simulink model "PubIfDecisionLSM_MDL"  (R2020b)
settings: configuration reference "DspaceConfig" (kept outside this file)
PostLoadFcn:
  | if any(exist('dsrtsu_mdlpostloadfcn', 'file') ~= 0), dsrtsu_mdlpostloadfcn('Execute', bdroot); end
InitFcn:
  | , if any(exist('rtifpga_mdlclblib', 'file') ~= 0), rtifpga_mdlclblib('Init', bdroot); end,
  | , if any(exist('dsmpb_private', 'file') ~= 0), dsmpb_private('dsmpb_mdlclblib', 'Init', bdroot); end,
values from neighbouring files (symbols this model uses):
  P_LSM_ALC_Enable = 0.0    [LSM_Parameter.sldd]
  P_LSM_AwayEdge_offset = 0.1    [LSM_Parameter.sldd]
  P_LSM_CentValidErr = 1.0    [LSM_Parameter.sldd]
  P_LSM_DOP_C0_EN_Limit = 0.8    [LSM_Parameter.sldd]
  P_LSM_DOP_C0_out_Limit = 2.0    [LSM_Parameter.sldd]
  P_LSM_DOP_C1_EN_Limit : value not decoded    [LSM_Parameter.sldd]
  P_LSM_DOP_C1_out_Limit : value not decoded    [LSM_Parameter.sldd]
  P_LSM_DOP_C1AndC2_Lim_X : value not decoded    [LSM_Parameter.sldd]
  P_LSM_DOP_C2_EN_Limit : value not decoded    [LSM_Parameter.sldd]
  P_LSM_DOP_C2_out_Limit : value not decoded    [LSM_Parameter.sldd]
  P_LSM_DOP_In_Pre2Dop_Dis = 1.0    [LSM_Parameter.sldd]
  P_LSM_DOP_Out_Pre2Dop_Dis = 2.0    [LSM_Parameter.sldd]
  P_LSM_DOP_PreDis_X : value not decoded    [LSM_Parameter.sldd]
  P_LSM_DOP_PreDis_Y : value not decoded    [LSM_Parameter.sldd]
  P_LSM_DOPEnableSW = 1.0    [LSM_Parameter.sldd]
  P_LSM_DOPValid_CheckTime = 0.06    [LSM_Parameter.sldd]
  P_LSM_DoubleLine_Curr2Cent_Dislimit = 0.5    [LSM_Parameter.sldd]
  P_LSM_DoubleLine_Dop2Cent_Dislimit = 0.5    [LSM_Parameter.sldd]
  P_LSM_DoubleLine_DOPOut_C1 : value not decoded    [LSM_Parameter.sldd]
  P_LSM_DoubleLine_Pre2Cent_Dislimit = 1.0    [LSM_Parameter.sldd]
  P_LSM_Error_Limit = 0.5    [LSM_Parameter.sldd]
  P_LSM_IFV2CenterAxis = 0.0    [LSM_Parameter.sldd]
  P_LSM_IFV2RearAxis = 0.0    [LSM_Parameter.sldd]
  P_LSM_Line2Edge_limit = 0.5    [LSM_Parameter.sldd]
  P_LSM_Line_Error = 0.1    [LSM_Parameter.sldd]
  P_LSM_LineSTD_Limit = 0.15    [LSM_Parameter.sldd]
  P_LSM_NOH_Switch = 0.0    [LSM_Parameter.sldd]
  P_LSM_OTL_C0_Factor = 1.0    [LSM_Parameter.sldd]
  P_LSM_OTL_C1_Factor = 0.5    [LSM_Parameter.sldd]
  P_LSM_OTL_C2_Factor = 0.5    [LSM_Parameter.sldd]
  P_LSM_Pre2OnlyLineDis = 5.0    [LSM_Parameter.sldd]
  P_LSM_Pre_t = 0.0    [LSM_Parameter.sldd]
  P_LSM_SingleLine_Cent2Edge_Dislimit = 100.0    [LSM_Parameter.sldd]
  P_LSM_SingleLine_Curr2Cent_Dislimit = 0.2    [LSM_Parameter.sldd]
  P_LSM_SingleLine_Dop2Cent_Dislimit = 0.2    [LSM_Parameter.sldd]
  P_LSM_SingleLine_DOPOut_C1 : value not decoded    [LSM_Parameter.sldd]
  P_LSM_SingleLine_Pre2Cent_Dislimit = 0.5    [LSM_Parameter.sldd]
  P_LSM_TJALimitSpd = 60.0    [LSM_Parameter.sldd]
undefined symbols (not defined in the file or in its folder): P_lCS_IFV2CenterAxis, P_LCS_IFV2RearAxis, P_LSM_EntryEdge_offset, P_LSM_EntryLnChngEnSwitch, P_LSM_EntryVanishDis, P_LSM_LinetLostTime, P_LSM_LineWijCal_C12, P_LSM_LineWijCal_C13, P_LSM_MapValid_ErrorSwitch, P_LSM_PosLineLcFac, P_LSM_SpdLim_Stub_Spd, P_LSM_SpdLim_StubLength, P_LSM_SpdTurnAlarm
libraries: simulink x324, TrueDurationTime x11
(part 14 of 25)

== system PubIfDecisionLSM_MDL/Subsystem1/TargetLineCalc_20ms/TargetLineCalc/Subsystem3/Subsystem2/Subsystem10 ==
  u : Inport
  MATLAB Function14 : MATLAB Function  TreatAsAtomicUnit=on
  Unit Delay : UnitDelay  SampleTime=-1  HasFrameUpgradeWarning=on
  y : Outport
  wires:
  MATLAB Function14/2(i) -> Unit Delay/1
  u/1 -> MATLAB Function14/1(u)
  Unit Delay/1 -> MATLAB Function14/2(i_k)
  MATLAB Function14/1(y) -> y/1

== system PubIfDecisionLSM_MDL/Subsystem1/TargetLineCalc_20ms/TargetLineCalc/Subsystem3/Subsystem2/Subsystem11 ==
  u : Inport
  MATLAB Function14 : MATLAB Function  TreatAsAtomicUnit=on
  Unit Delay : UnitDelay  SampleTime=-1  HasFrameUpgradeWarning=on
  y : Outport
  wires:
  MATLAB Function14/1(y) -> y/1
  Unit Delay/1 -> MATLAB Function14/2(i_k)
  u/1 -> MATLAB Function14/1(u)
  MATLAB Function14/2(i) -> Unit Delay/1

== system PubIfDecisionLSM_MDL/Subsystem1/TargetLineCalc_20ms/TargetLineCalc/Subsystem3/Subsystem2/Subsystem12 ==
  u : Inport
  MATLAB Function14 : MATLAB Function  TreatAsAtomicUnit=on
  Unit Delay : UnitDelay  SampleTime=-1  HasFrameUpgradeWarning=on
  y : Outport
  wires:
  MATLAB Function14/2(i) -> Unit Delay/1
  u/1 -> MATLAB Function14/1(u)
  Unit Delay/1 -> MATLAB Function14/2(i_k)
  MATLAB Function14/1(y) -> y/1

== system PubIfDecisionLSM_MDL/Subsystem1/TargetLineCalc_20ms/TargetLineCalc/Subsystem3/Subsystem2/Subsystem13 ==
  u : Inport
  MATLAB Function14 : MATLAB Function  TreatAsAtomicUnit=on
  Unit Delay : UnitDelay  SampleTime=-1  HasFrameUpgradeWarning=on
  y : Outport
  wires:
  MATLAB Function14/2(i) -> Unit Delay/1
  u/1 -> MATLAB Function14/1(u)
  Unit Delay/1 -> MATLAB Function14/2(i_k)
  MATLAB Function14/1(y) -> y/1

== system PubIfDecisionLSM_MDL/Subsystem1/TargetLineCalc_20ms/TargetLineCalc/Subsystem3/Subsystem2/Subsystem14 ==
  u : Inport
  MATLAB Function14 : MATLAB Function  TreatAsAtomicUnit=on
  Unit Delay : UnitDelay  SampleTime=-1  HasFrameUpgradeWarning=on
  y : Outport
  wires:
  MATLAB Function14/1(y) -> y/1
  Unit Delay/1 -> MATLAB Function14/2(i_k)
  u/1 -> MATLAB Function14/1(u)
  MATLAB Function14/2(i) -> Unit Delay/1

== system PubIfDecisionLSM_MDL/Subsystem1/TargetLineCalc_20ms/TargetLineCalc/Subsystem3/Subsystem2/Subsystem15 ==
  u : Inport
  MATLAB Function14 : MATLAB Function  TreatAsAtomicUnit=on
  Unit Delay : UnitDelay  SampleTime=-1  HasFrameUpgradeWarning=on
  y : Outport
  wires:
  MATLAB Function14/1(y) -> y/1
  Unit Delay/1 -> MATLAB Function14/2(i_k)
  u/1 -> MATLAB Function14/1(u)
  MATLAB Function14/2(i) -> Unit Delay/1

== system PubIfDecisionLSM_MDL/Subsystem1/TargetLineCalc_20ms/TargetLineCalc/Subsystem3/Subsystem2/Subsystem16 ==
  u : Inport
  MATLAB Function14 : MATLAB Function  TreatAsAtomicUnit=on
  Unit Delay : UnitDelay  SampleTime=-1  HasFrameUpgradeWarning=on
  y : Outport
  wires:
  MATLAB Function14/2(i) -> Unit Delay/1
  u/1 -> MATLAB Function14/1(u)
  Unit Delay/1 -> MATLAB Function14/2(i_k)
  MATLAB Function14/1(y) -> y/1

== system PubIfDecisionLSM_MDL/Subsystem1/TargetLineCalc_20ms/TargetLineCalc/Subsystem3/Subsystem2/Subsystem2 ==
  u : Inport
  MATLAB Function14 : MATLAB Function  TreatAsAtomicUnit=on
  Unit Delay : UnitDelay  SampleTime=-1  HasFrameUpgradeWarning=on
  y : Outport
  wires:
  MATLAB Function14/1(y) -> y/1
  Unit Delay/1 -> MATLAB Function14/2(i_k)
  u/1 -> MATLAB Function14/1(u)
  MATLAB Function14/2(i) -> Unit Delay/1

== system PubIfDecisionLSM_MDL/Subsystem1/TargetLineCalc_20ms/TargetLineCalc/Subsystem3/Subsystem2/Subsystem3 ==
  u : Inport
  MATLAB Function14 : MATLAB Function  TreatAsAtomicUnit=on
  Unit Delay : UnitDelay  SampleTime=-1  HasFrameUpgradeWarning=on
  y : Outport
  wires:
  MATLAB Function14/2(i) -> Unit Delay/1
  u/1 -> MATLAB Function14/1(u)
  Unit Delay/1 -> MATLAB Function14/2(i_k)
  MATLAB Function14/1(y) -> y/1

== system PubIfDecisionLSM_MDL/Subsystem1/TargetLineCalc_20ms/TargetLineCalc/Subsystem3/Subsystem2/Subsystem4 ==
  u : Inport
  MATLAB Function14 : MATLAB Function  TreatAsAtomicUnit=on
  Unit Delay : UnitDelay  SampleTime=-1  HasFrameUpgradeWarning=on
  y : Outport
  wires:
  MATLAB Function14/1(y) -> y/1
  Unit Delay/1 -> MATLAB Function14/2(i_k)
  u/1 -> MATLAB Function14/1(u)
  MATLAB Function14/2(i) -> Unit Delay/1

== system PubIfDecisionLSM_MDL/Subsystem1/TargetLineCalc_20ms/TargetLineCalc/Subsystem3/Subsystem2/Subsystem5 ==
  u : Inport
  MATLAB Function14 : MATLAB Function  TreatAsAtomicUnit=on
  Unit Delay : UnitDelay  SampleTime=-1  HasFrameUpgradeWarning=on
  y : Outport
  wires:
  MATLAB Function14/1(y) -> y/1
  Unit Delay/1 -> MATLAB Function14/2(i_k)
  u/1 -> MATLAB Function14/1(u)
  MATLAB Function14/2(i) -> Unit Delay/1

== system PubIfDecisionLSM_MDL/Subsystem1/TargetLineCalc_20ms/TargetLineCalc/Subsystem3/Subsystem2/Subsystem6 ==
  u : Inport
  MATLAB Function14 : MATLAB Function  TreatAsAtomicUnit=on
  Unit Delay : UnitDelay  SampleTime=-1  HasFrameUpgradeWarning=on
  y : Outport
  wires:
  MATLAB Function14/2(i) -> Unit Delay/1
  u/1 -> MATLAB Function14/1(u)
  Unit Delay/1 -> MATLAB Function14/2(i_k)
  MATLAB Function14/1(y) -> y/1

== system PubIfDecisionLSM_MDL/Subsystem1/TargetLineCalc_20ms/TargetLineCalc/Subsystem3/Subsystem2/Subsystem7 ==
  u : Inport
  MATLAB Function14 : MATLAB Function  TreatAsAtomicUnit=on
  Unit Delay : UnitDelay  SampleTime=-1  HasFrameUpgradeWarning=on
  y : Outport
  wires:
  MATLAB Function14/1(y) -> y/1
  Unit Delay/1 -> MATLAB Function14/2(i_k)
  u/1 -> MATLAB Function14/1(u)
  MATLAB Function14/2(i) -> Unit Delay/1

== system PubIfDecisionLSM_MDL/Subsystem1/TargetLineCalc_20ms/TargetLineCalc/Subsystem3/Subsystem2/Subsystem8 ==
  u : Inport
  MATLAB Function14 : MATLAB Function  TreatAsAtomicUnit=on
  Unit Delay : UnitDelay  SampleTime=-1  HasFrameUpgradeWarning=on
  y : Outport
  wires:
  MATLAB Function14/2(i) -> Unit Delay/1
  u/1 -> MATLAB Function14/1(u)
  Unit Delay/1 -> MATLAB Function14/2(i_k)
  MATLAB Function14/1(y) -> y/1

== system PubIfDecisionLSM_MDL/Subsystem1/TargetLineCalc_20ms/TargetLineCalc/Subsystem3/Subsystem2/Subsystem9 ==
  u : Inport
  MATLAB Function14 : MATLAB Function  TreatAsAtomicUnit=on
  Unit Delay : UnitDelay  SampleTime=-1  HasFrameUpgradeWarning=on
  y : Outport
  wires:
  MATLAB Function14/1(y) -> y/1
  Unit Delay/1 -> MATLAB Function14/2(i_k)
  u/1 -> MATLAB Function14/1(u)
  MATLAB Function14/2(i) -> Unit Delay/1

== system PubIfDecisionLSM_MDL/Subsystem1/TargetLineCalc_20ms2/TargetLineCalc/Subsystem3/Subsystem/Subsystem ==
  count : Inport
  startDis1 : Inport  Port=2
  endDis1 : Inport  Port=3
  type1 : Inport  Port=4
  startDis2 : Inport  Port=5
  endDis2 : Inport  Port=6
  type2 : Inport  Port=7
  startDis3 : Inport  Port=8
  endDis3 : Inport  Port=9
  type3 : Inport  Port=10
  startDis4 : Inport  Port=11
  endDis4 : Inport  Port=12
  type4 : Inport  Port=13
  startDis5 : Inport  Port=14
  endDis5 : Inport  Port=15
  type5 : Inport  Port=16
  MATLAB Function : MATLAB Function  TreatAsAtomicUnit=on
  Mux : Mux  Inputs=5
  Mux1 : Mux  Inputs=5
  Mux2 : Mux  Inputs=5
  Terminator1 : Terminator
  LSM_PilotNohExitDist : Outport  OutDataTypeStr=uint16  PortDimensions=1  BusOutputAsStruct=on
  NoPUCR : Outport  Port=2
  NoPUCR_Dis : Outport  Port=3
  wires:
  count/1 -> MATLAB Function/1(count)
  MATLAB Function/1(PilotNohExitDist) -> LSM_PilotNohExitDist/1
  Mux2/1 -> MATLAB Function/3(type)
  Mux1/1 -> Terminator1/1
  Mux/1 -> MATLAB Function/2(startDis)
  type5/1 -> Mux2/5
  type4/1 -> Mux2/4
  type3/1 -> Mux2/3
  type2/1 -> Mux2/2
  type1/1 -> Mux2/1
  endDis4/1 -> Mux1/4
  endDis5/1 -> Mux1/5
  endDis3/1 -> Mux1/3
  endDis2/1 -> Mux1/2
  endDis1/1 -> Mux1/1
  startDis5/1 -> Mux/5
  startDis4/1 -> Mux/4
  startDis3/1 -> Mux/3
  startDis2/1 -> Mux/2
  startDis1/1 -> Mux/1
  MATLAB Function/2(NoPUCR) -> NoPUCR/1
  MATLAB Function/3(NoPUCR_Dis) -> NoPUCR_Dis/1

== system PubIfDecisionLSM_MDL/Subsystem1/TargetLineCalc_20ms2/TargetLineCalc/Subsystem3/Subsystem1/Subsystem ==
  u : Inport
  NoPUCR : Inport  Port=2
  Chart : Stateflow chart  TreatAsAtomicUnit=on
      settings: PortSchema="{\"entries\":[{\"content\":{\"sides\":[{\"content\":{\"connectorIds\":[\"In2\",\"In3\",\"In1\"]},\"type\":\"ConnectorPlacement.EquallySpacedRectSide\",\"uuid\":\"5c1eee58-4a30-4b86-84c5-00e679bbbe27\"},{\"content\":{\"connectorIds\":[\"Out1\"],\"side\":\"RIGHT\"},\"type\":\"ConnectorPlacement.EquallySpacedRectSide\",\"uuid\":\"5608aa44-0f6f-4814-b65d-f19ffe57378f\"},{\"content\":{\"connectorIds\":[],\"side\":\"TOP\"},\"type\":\"ConnectorPlacement.EquallySpacedRectSide\",\"uuid\":\"e8d8f265-698a-4610-8e00-f2739970e5c8\"},{\"content\":{\"connectorIds\":[],\"side\":\"HIDDEN\"},\"type\":\"ConnectorPlacement.EquallySpacedRectSide\",\"uuid\":\"a29265fa-427e-416e-86d2-9419d10abf4c\"}]},\"type\":\"ConnectorPlacement.EquallySpacedConnector\",\"uuid\":\"6539a137-c87a-4ed7-8d33-ef009a5dd0dc\"}],\"packageUris\":[\"http://schema.mathworks.com/mf0/Connector/R2020b\"],\"version\":\"1.0\"}"
  MATLAB Function1 : MATLAB Function  TreatAsAtomicUnit=on
  Unit Delay1 : UnitDelay  SampleTime=-1  HasFrameUpgradeWarning=on
  Unit Delay10 : UnitDelay  SampleTime=-1  HasFrameUpgradeWarning=on
  Unit Delay11 : UnitDelay  SampleTime=-1  HasFrameUpgradeWarning=on
  y : Outport
  wires:
  Unit Delay1/1 -> Chart/3(nav_pathK)
  Chart/1(y) -> y/1
  NoPUCR/1 -> Chart/1(NoPUCR)
  u/1 -> MATLAB Function1/1(u), Unit Delay10/1
  MATLAB Function1/2(count) -> Unit Delay11/1
  Unit Delay10/1 -> MATLAB Function1/2(uK)
  Unit Delay11/1 -> MATLAB Function1/3(countK)
  MATLAB Function1/1(y) -> Chart/2(nav_path), Unit Delay1/1

== system PubIfDecisionLSM_MDL/Subsystem1/TargetLineCalc_20ms2/TargetLineCalc/Subsystem3/Subsystem2/Subsystem ==
  In1 : Inport
  MATLAB Function4 : MATLAB Function  TreatAsAtomicUnit=on
  Unit Delay : UnitDelay  SampleTime=-1  HasFrameUpgradeWarning=on
  Unit Delay2 : UnitDelay  SampleTime=-1  HasFrameUpgradeWarning=on
  y : Outport
  wires:
  In1/1 -> Unit Delay/1, MATLAB Function4/1(u)
  Unit Delay/1 -> MATLAB Function4/2(uK)
  MATLAB Function4/1(y) -> y/1
  MATLAB Function4/2(i) -> Unit Delay2/1
  Unit Delay2/1 -> MATLAB Function4/3(iK)

== system PubIfDecisionLSM_MDL/Subsystem1/TargetLineCalc_20ms2/TargetLineCalc/Subsystem3/Subsystem2/Subsystem1 ==
  In1 : Inport
  MATLAB Function4 : MATLAB Function  TreatAsAtomicUnit=on
  Unit Delay : UnitDelay  SampleTime=-1  HasFrameUpgradeWarning=on
  Unit Delay2 : UnitDelay  SampleTime=-1  HasFrameUpgradeWarning=on
  y : Outport
  wires:
  Unit Delay2/1 -> MATLAB Function4/3(iK)
  MATLAB Function4/2(i) -> Unit Delay2/1
  MATLAB Function4/1(y) -> y/1
  Unit Delay/1 -> MATLAB Function4/2(uK)
  In1/1 -> MATLAB Function4/1(u), Unit Delay/1

== system PubIfDecisionLSM_MDL/Subsystem1/TargetLineCalc_20ms2/TargetLineCalc/Subsystem3/Subsystem2/Subsystem10 ==
  laneValid : Inport
  u : Inport  Port=2
  AND : Logic  Inputs=5  AllPortsSameDT=off  OutDataTypeStr=boolean
  Compare To Constant{1..4,26} (5 alike) : simulink/Logic and Bit Operations/Compare To Constant  relop=>  const=1.8  OutDataTypeStr=boolean
  Compare To Constant{5..9} (5 alike) : simulink/Logic and Bit Operations/Compare To Constant  relop=<  const=-1.8  OutDataTypeStr=boolean
  Constant : Constant  Value=0  OutDataTypeStr=boolean
  OR{,1..4} (5 alike) : Logic  Operator=OR  AllPortsSameDT=off  OutDataTypeStr=boolean
  Switch : Switch  Criteria=u2 > Threshold
  Unit Delay{1..4} (4 alike) : UnitDelay  SampleTime=-1  HasFrameUpgradeWarning=on
  y : Outport
  wires:
  u/1 -> Unit Delay1/1, Compare To Constant5/1, Compare To Constant26/1
  Unit Delay1/1 -> Unit Delay2/1, Compare To Constant6/1, Compare To Constant1/1
  Unit Delay2/1 -> Compare To Constant7/1, Compare To Constant2/1, Unit Delay3/1
  Unit Delay3/1 -> Compare To Constant3/1, Compare To Constant8/1, Unit Delay4/1
  Unit Delay4/1 -> Compare To Constant9/1, Compare To Constant4/1
  Compare To Constant26/1 -> OR/2
  Compare To Constant1/1 -> OR1/2
  Compare To Constant2/1 -> OR2/2
  Compare To Constant3/1 -> OR3/2
  Compare To Constant4/1 -> OR4/2
  laneValid/1 -> Switch/2
  AND/1 -> Switch/1
  Switch/1 -> y/1
  Constant/1 -> Switch/3
  Compare To Constant5/1 -> OR/1
  OR/1 -> AND/1
  Compare To Constant6/1 -> OR1/1
  OR1/1 -> AND/2
  Compare To Constant7/1 -> OR2/1
  OR2/1 -> AND/3
  Compare To Constant8/1 -> OR3/1
  OR3/1 -> AND/4
  Compare To Constant9/1 -> OR4/1
  OR4/1 -> AND/5

== system PubIfDecisionLSM_MDL/Subsystem1/TargetLineCalc_20ms2/TargetLineCalc/Subsystem3/Subsystem2/Subsystem17 ==
  b_is_available : Inport
  Entry_bIsLineExist : Inport  Port=2
  MATLAB Function1 : MATLAB Function  TreatAsAtomicUnit=on
  Unit Delay : UnitDelay  SampleTime=-1  HasFrameUpgradeWarning=on
  Unit Delay1 : UnitDelay  SampleTime=-1  HasFrameUpgradeWarning=on
  Unit Delay2 : UnitDelay  SampleTime=-1  HasFrameUpgradeWarning=on
  enStubExist : Outport
  wires:
  Unit Delay2/1 -> MATLAB Function1/5(enStubExistK)
  MATLAB Function1/1(enStubExist) -> enStubExist/1, Unit Delay2/1
  b_is_available/1 -> MATLAB Function1/1(b_is_available), Unit Delay/1
  Entry_bIsLineExist/1 -> MATLAB Function1/3(Entry_bIsLineExist), Unit Delay1/1
  Unit Delay/1 -> MATLAB Function1/2(b_is_availableK)
  Unit Delay1/1 -> MATLAB Function1/4(Entry_bIsLineExistK)

== system PubIfDecisionLSM_MDL/Subsystem1/TargetLineCalc_20ms2/TargetLineCalc/Subsystem3/Subsystem2/Subsystem19 ==
  laneValid : Inport
  u : Inport  Port=2
  AND : Logic  Inputs=5  AllPortsSameDT=off  OutDataTypeStr=boolean
  Compare To Constant{1..4,26} (5 alike) : simulink/Logic and Bit Operations/Compare To Constant  relop=>  const=1.8  OutDataTypeStr=boolean
  Compare To Constant{5..9} (5 alike) : simulink/Logic and Bit Operations/Compare To Constant  relop=<  const=-1.8  OutDataTypeStr=boolean
  Constant : Constant  Value=0  OutDataTypeStr=boolean
  OR{,1..4} (5 alike) : Logic  Operator=OR  AllPortsSameDT=off  OutDataTypeStr=boolean
  Switch : Switch  Criteria=u2 > Threshold
  Unit Delay{1..4} (4 alike) : UnitDelay  SampleTime=-1  HasFrameUpgradeWarning=on
  y : Outport
  wires:
  u/1 -> Unit Delay1/1, Compare To Constant5/1, Compare To Constant26/1
  Unit Delay1/1 -> Unit Delay2/1, Compare To Constant6/1, Compare To Constant1/1
  Unit Delay2/1 -> Compare To Constant7/1, Compare To Constant2/1, Unit Delay3/1
  Unit Delay3/1 -> Compare To Constant3/1, Compare To Constant8/1, Unit Delay4/1
  Unit Delay4/1 -> Compare To Constant9/1, Compare To Constant4/1
  Compare To Constant26/1 -> OR/2
  Compare To Constant1/1 -> OR1/2
  Compare To Constant2/1 -> OR2/2
  Compare To Constant3/1 -> OR3/2
  Compare To Constant4/1 -> OR4/2
  laneValid/1 -> Switch/2
  AND/1 -> Switch/1
  Switch/1 -> y/1
  Constant/1 -> Switch/3
  Compare To Constant5/1 -> OR/1
  OR/1 -> AND/1
  Compare To Constant6/1 -> OR1/1
  OR1/1 -> AND/2
  Compare To Constant7/1 -> OR2/1
  OR2/1 -> AND/3
  Compare To Constant8/1 -> OR3/1
  OR3/1 -> AND/4
  Compare To Constant9/1 -> OR4/1
  OR4/1 -> AND/5

== system PubIfDecisionLSM_MDL/Subsystem1/TargetLineCalc_20ms2/TargetLineCalc/Subsystem3/Subsystem2/Subsystem2 ==
  laneValid : Inport
  u : Inport  Port=2
  MATLAB Function14 : MATLAB Function  TreatAsAtomicUnit=on
  Unit Delay{,1..6} (7 alike) : UnitDelay  SampleTime=-1  HasFrameUpgradeWarning=on
  y : Outport
  wires:
  MATLAB Function14/3(y_store) -> Unit Delay2/1
  MATLAB Function14/1(y) -> y/1
  Unit Delay/1 -> MATLAB Function14/5(countK1)
  laneValid/1 -> Unit Delay3/1, MATLAB Function14/1(laneValid)
  u/1 -> Unit Delay1/1, MATLAB Function14/3(u)
  MATLAB Function14/2(count1) -> Unit Delay/1
  Unit Delay1/1 -> MATLAB Function14/4(uK)
  Unit Delay2/1 -> MATLAB Function14/6(y_storeK)
  MATLAB Function14/4(timeValid1) -> Unit Delay4/1
  Unit Delay4/1 -> MATLAB Function14/7(timeValidK1)
  Unit Delay3/1 -> MATLAB Function14/2(laneValidK)
  MATLAB Function14/5(count2) -> Unit Delay5/1
  Unit Delay5/1 -> MATLAB Function14/8(countK2)
  MATLAB Function14/6(timeValid2) -> Unit Delay6/1
  Unit Delay6/1 -> MATLAB Function14/9(timeValidK2)

== system PubIfDecisionLSM_MDL/Subsystem1/TargetLineCalc_20ms2/TargetLineCalc/Subsystem3/Subsystem2/Subsystem3 ==
  laneValid : Inport
  u : Inport  Port=2
  AND : Logic  Inputs=5  AllPortsSameDT=off  OutDataTypeStr=boolean
  Compare To Constant{1..4,26} (5 alike) : simulink/Logic and Bit Operations/Compare To Constant  relop=>  const=1.8  OutDataTypeStr=boolean
  Compare To Constant{5..9} (5 alike) : simulink/Logic and Bit Operations/Compare To Constant  relop=<  const=-1.8  OutDataTypeStr=boolean
  Constant : Constant  Value=0  OutDataTypeStr=boolean
  OR{,1..4} (5 alike) : Logic  Operator=OR  AllPortsSameDT=off  OutDataTypeStr=boolean
  Switch : Switch  Criteria=u2 > Threshold
  Unit Delay{1..4} (4 alike) : UnitDelay  SampleTime=-1  HasFrameUpgradeWarning=on
  y : Outport
  wires:
  u/1 -> Unit Delay1/1, Compare To Constant5/1, Compare To Constant26/1
  Unit Delay1/1 -> Unit Delay2/1, Compare To Constant6/1, Compare To Constant1/1
  Unit Delay2/1 -> Compare To Constant7/1, Compare To Constant2/1, Unit Delay3/1
  Unit Delay3/1 -> Compare To Constant3/1, Compare To Constant8/1, Unit Delay4/1
  Unit Delay4/1 -> Compare To Constant9/1, Compare To Constant4/1
  Compare To Constant26/1 -> OR/2
  Compare To Constant1/1 -> OR1/2
  Compare To Constant2/1 -> OR2/2
  Compare To Constant3/1 -> OR3/2
  Compare To Constant4/1 -> OR4/2
  laneValid/1 -> Switch/2
  AND/1 -> Switch/1
  Switch/1 -> y/1
  Constant/1 -> Switch/3
  Compare To Constant5/1 -> OR/1
  OR/1 -> AND/1
  Compare To Constant6/1 -> OR1/1
  OR1/1 -> AND/2
  Compare To Constant7/1 -> OR2/1
  OR2/1 -> AND/3
  Compare To Constant8/1 -> OR3/1
  OR3/1 -> AND/4
  Compare To Constant9/1 -> OR4/1
  OR4/1 -> AND/5

== system PubIfDecisionLSM_MDL/Subsystem1/TargetLineCalc_20ms2/TargetLineCalc/Subsystem3/Subsystem2/Subsystem4 ==
  laneValid : Inport
  u : Inport  Port=2
  AND : Logic  Inputs=5  AllPortsSameDT=off  OutDataTypeStr=boolean
  Compare To Constant{1..4,26} (5 alike) : simulink/Logic and Bit Operations/Compare To Constant  relop=>  const=1.8  OutDataTypeStr=boolean
  Compare To Constant{5..9} (5 alike) : simulink/Logic and Bit Operations/Compare To Constant  relop=<  const=-1.8  OutDataTypeStr=boolean
  Constant : Constant  Value=0  OutDataTypeStr=boolean
  OR{,1..4} (5 alike) : Logic  Operator=OR  AllPortsSameDT=off  OutDataTypeStr=boolean
  Switch : Switch  Criteria=u2 > Threshold
  Unit Delay{1..4} (4 alike) : UnitDelay  SampleTime=-1  HasFrameUpgradeWarning=on
  y : Outport
  wires:
  OR4/1 -> AND/5
  Compare To Constant9/1 -> OR4/1
  OR3/1 -> AND/4
  Compare To Constant8/1 -> OR3/1
  OR2/1 -> AND/3
  Compare To Constant7/1 -> OR2/1
  OR1/1 -> AND/2
  Compare To Constant6/1 -> OR1/1
  OR/1 -> AND/1
  Compare To Constant5/1 -> OR/1
  Constant/1 -> Switch/3
  Switch/1 -> y/1
  AND/1 -> Switch/1
  laneValid/1 -> Switch/2
  Compare To Constant4/1 -> OR4/2
  Compare To Constant3/1 -> OR3/2
  Compare To Constant2/1 -> OR2/2
  Compare To Constant1/1 -> OR1/2
  Compare To Constant26/1 -> OR/2
  Unit Delay4/1 -> Compare To Constant4/1, Compare To Constant9/1
  Unit Delay3/1 -> Unit Delay4/1, Compare To Constant8/1, Compare To Constant3/1
  Unit Delay2/1 -> Unit Delay3/1, Compare To Constant2/1, Compare To Constant7/1
  Unit Delay1/1 -> Compare To Constant1/1, Compare To Constant6/1, Unit Delay2/1
  u/1 -> Compare To Constant26/1, Compare To Constant5/1, Unit Delay1/1

== system PubIfDecisionLSM_MDL/Subsystem1/TargetLineCalc_20ms2/TargetLineCalc/Subsystem3/Subsystem2/Subsystem5 ==
  laneValid : Inport
  u : Inport  Port=2
  AND : Logic  Inputs=5  AllPortsSameDT=off  OutDataTypeStr=boolean
  Compare To Constant{1..4,26} (5 alike) : simulink/Logic and Bit Operations/Compare To Constant  relop=>  const=1.8  OutDataTypeStr=boolean
  Compare To Constant{5..9} (5 alike) : simulink/Logic and Bit Operations/Compare To Constant  relop=<  const=-1.8  OutDataTypeStr=boolean
  Constant : Constant  Value=0  OutDataTypeStr=boolean
  OR{,1..4} (5 alike) : Logic  Operator=OR  AllPortsSameDT=off  OutDataTypeStr=boolean
  Switch : Switch  Criteria=u2 > Threshold
  Unit Delay{1..4} (4 alike) : UnitDelay  SampleTime=-1  HasFrameUpgradeWarning=on
  y : Outport
  wires:
  OR4/1 -> AND/5
  Compare To Constant9/1 -> OR4/1
  OR3/1 -> AND/4
  Compare To Constant8/1 -> OR3/1
  OR2/1 -> AND/3
  Compare To Constant7/1 -> OR2/1
  OR1/1 -> AND/2
  Compare To Constant6/1 -> OR1/1
  OR/1 -> AND/1
  Compare To Constant5/1 -> OR/1
  Constant/1 -> Switch/3
  Switch/1 -> y/1
  AND/1 -> Switch/1
  laneValid/1 -> Switch/2
  Compare To Constant4/1 -> OR4/2
  Compare To Constant3/1 -> OR3/2
  Compare To Constant2/1 -> OR2/2
  Compare To Constant1/1 -> OR1/2
  Compare To Constant26/1 -> OR/2
  Unit Delay4/1 -> Compare To Constant4/1, Compare To Constant9/1
  Unit Delay3/1 -> Unit Delay4/1, Compare To Constant8/1, Compare To Constant3/1
  Unit Delay2/1 -> Unit Delay3/1, Compare To Constant2/1, Compare To Constant7/1
  Unit Delay1/1 -> Compare To Constant1/1, Compare To Constant6/1, Unit Delay2/1
  u/1 -> Compare To Constant26/1, Compare To Constant5/1, Unit Delay1/1

== system PubIfDecisionLSM_MDL/Subsystem1/TargetLineCalc_20ms2/TargetLineCalc/Subsystem3/Subsystem2/Subsystem6 ==
  laneValid : Inport
  u : Inport  Port=2
  AND : Logic  Inputs=5  AllPortsSameDT=off  OutDataTypeStr=boolean
  Compare To Constant{1..4,26} (5 alike) : simulink/Logic and Bit Operations/Compare To Constant  relop=>  const=1.8  OutDataTypeStr=boolean
  Compare To Constant{5..9} (5 alike) : simulink/Logic and Bit Operations/Compare To Constant  relop=<  const=-1.8  OutDataTypeStr=boolean
  Constant : Constant  Value=0  OutDataTypeStr=boolean
  OR{,1..4} (5 alike) : Logic  Operator=OR  AllPortsSameDT=off  OutDataTypeStr=boolean
  Switch : Switch  Criteria=u2 > Threshold
  Unit Delay{1..4} (4 alike) : UnitDelay  SampleTime=-1  HasFrameUpgradeWarning=on
  y : Outport
  wires:
  u/1 -> Unit Delay1/1, Compare To Constant5/1, Compare To Constant26/1
  Unit Delay1/1 -> Unit Delay2/1, Compare To Constant6/1, Compare To Constant1/1
  Unit Delay2/1 -> Compare To Constant7/1, Compare To Constant2/1, Unit Delay3/1
  Unit Delay3/1 -> Compare To Constant3/1, Compare To Constant8/1, Unit Delay4/1
  Unit Delay4/1 -> Compare To Constant9/1, Compare To Constant4/1
  Compare To Constant26/1 -> OR/2
  Compare To Constant1/1 -> OR1/2
  Compare To Constant2/1 -> OR2/2
  Compare To Constant3/1 -> OR3/2
  Compare To Constant4/1 -> OR4/2
  laneValid/1 -> Switch/2
  AND/1 -> Switch/1
  Switch/1 -> y/1
  Constant/1 -> Switch/3
  Compare To Constant5/1 -> OR/1
  OR/1 -> AND/1
  Compare To Constant6/1 -> OR1/1
  OR1/1 -> AND/2
  Compare To Constant7/1 -> OR2/1
  OR2/1 -> AND/3
  Compare To Constant8/1 -> OR3/1
  OR3/1 -> AND/4
  Compare To Constant9/1 -> OR4/1
  OR4/1 -> AND/5

== system PubIfDecisionLSM_MDL/Subsystem1/TargetLineCalc_20ms2/TargetLineCalc/Subsystem3/Subsystem2/Subsystem8 ==
  laneValid : Inport
  u : Inport  Port=2
  AND : Logic  Inputs=5  AllPortsSameDT=off  OutDataTypeStr=boolean
  Compare To Constant{1..4,26} (5 alike) : simulink/Logic and Bit Operations/Compare To Constant  relop=>  const=1.8  OutDataTypeStr=boolean
  Compare To Constant{5..9} (5 alike) : simulink/Logic and Bit Operations/Compare To Constant  relop=<  const=-1.8  OutDataTypeStr=boolean
  Constant : Constant  Value=0  OutDataTypeStr=boolean
  OR{,1..4} (5 alike) : Logic  Operator=OR  AllPortsSameDT=off  OutDataTypeStr=boolean
  Switch : Switch  Criteria=u2 > Threshold
  Unit Delay{1..4} (4 alike) : UnitDelay  SampleTime=-1  HasFrameUpgradeWarning=on
  y : Outport
  wires:
  OR4/1 -> AND/5
  Compare To Constant9/1 -> OR4/1
  OR3/1 -> AND/4
  Compare To Constant8/1 -> OR3/1
  OR2/1 -> AND/3
  Compare To Constant7/1 -> OR2/1
  OR1/1 -> AND/2
  Compare To Constant6/1 -> OR1/1
  OR/1 -> AND/1
  Compare To Constant5/1 -> OR/1
  Constant/1 -> Switch/3
  Switch/1 -> y/1
  AND/1 -> Switch/1
  laneValid/1 -> Switch/2
  Compare To Constant4/1 -> OR4/2
  Compare To Constant3/1 -> OR3/2
  Compare To Constant2/1 -> OR2/2
  Compare To Constant1/1 -> OR1/2
  Compare To Constant26/1 -> OR/2
  Unit Delay4/1 -> Compare To Constant4/1, Compare To Constant9/1
  Unit Delay3/1 -> Unit Delay4/1, Compare To Constant8/1, Compare To Constant3/1
  Unit Delay2/1 -> Unit Delay3/1, Compare To Constant2/1, Compare To Constant7/1
  Unit Delay1/1 -> Compare To Constant1/1, Compare To Constant6/1, Unit Delay2/1
  u/1 -> Compare To Constant26/1, Compare To Constant5/1, Unit Delay1/1

== system PubIfDecisionLSM_MDL/Subsystem1/TargetLineCalc_20ms2/TargetLineCalc/Subsystem3/Subsystem2/Subsystem9 ==
  laneValid : Inport
  u : Inport  Port=2
  AND : Logic  Inputs=5  AllPortsSameDT=off  OutDataTypeStr=boolean
  Compare To Constant{1..4,26} (5 alike) : simulink/Logic and Bit Operations/Compare To Constant  relop=>  const=1.8  OutDataTypeStr=boolean
  Compare To Constant{5..9} (5 alike) : simulink/Logic and Bit Operations/Compare To Constant  relop=<  const=-1.8  OutDataTypeStr=boolean
  Constant : Constant  Value=0  OutDataTypeStr=boolean
  OR{,1..4} (5 alike) : Logic  Operator=OR  AllPortsSameDT=off  OutDataTypeStr=boolean
  Switch : Switch  Criteria=u2 > Threshold
  Unit Delay{1..4} (4 alike) : UnitDelay  SampleTime=-1  HasFrameUpgradeWarning=on
  y : Outport
  wires:
  OR4/1 -> AND/5
  Compare To Constant9/1 -> OR4/1
  OR3/1 -> AND/4
  Compare To Constant8/1 -> OR3/1
  OR2/1 -> AND/3
  Compare To Constant7/1 -> OR2/1
  OR1/1 -> AND/2
  Compare To Constant6/1 -> OR1/1
  OR/1 -> AND/1
  Compare To Constant5/1 -> OR/1
  Constant/1 -> Switch/3
  Switch/1 -> y/1
  AND/1 -> Switch/1
  laneValid/1 -> Switch/2
  Compare To Constant4/1 -> OR4/2
  Compare To Constant3/1 -> OR3/2
  Compare To Constant2/1 -> OR2/2
  Compare To Constant1/1 -> OR1/2
  Compare To Constant26/1 -> OR/2
  Unit Delay4/1 -> Compare To Constant4/1, Compare To Constant9/1
  Unit Delay3/1 -> Unit Delay4/1, Compare To Constant8/1, Compare To Constant3/1
  Unit Delay2/1 -> Unit Delay3/1, Compare To Constant2/1, Compare To Constant7/1
  Unit Delay1/1 -> Compare To Constant1/1, Compare To Constant6/1, Unit Delay2/1
  u/1 -> Compare To Constant26/1, Compare To Constant5/1, Unit Delay1/1

== matlab function PubIfDecisionLSM_MDL/Subsystem1/TargetLineCalc_20ms/TargetLineCalc/LREWidthCalc ==
  data: LRELineConf input uint8 size=2; a1 input single size=2; a0 input single size=2; LRELineUpdate input boolean size=1; LREWidthK1 input single size=1; LREWidth output single size=1
function LREWidth  = VisRoadWidth(LRELineConf,a1,a0,LRELineUpdate,LREWidthK1)

LREWidth = LREWidthK1;
Update = false;
temp = single(0);

if LRELineUpdate
    if (LRELineConf(1)>0)&&(LRELineConf(2)>0)
        if abs(57.3*(atan(a1(1)) - atan(a1(2))))<3
            temp = (a0(1) - a0(2))/sqrt(a1(2)^2 + single(1));
            Update = true;
        end
    end
    if Update
        LREWidth = 0.1*(temp - LREWidthK1) + LREWidthK1;
    end
end

== matlab function PubIfDecisionLSM_MDL/Subsystem1/TargetLineCalc_20ms/TargetLineCalc/MATLAB Function ==
  data: Cur_avail input; MrcStopLane output; Cur_LaneType input; Right_avail input
function MrcStopLane = fcn(Cur_avail,Cur_LaneType,Right_avail)
MrcStopLane = uint8(0);
if (Cur_avail>0&&Cur_LaneType==5)||(Cur_avail>0&&Cur_LaneType~=5&&Right_avail==0)
    MrcStopLane = uint8(1);
end

== matlab function PubIfDecisionLSM_MDL/Subsystem1/TargetLineCalc_20ms/TargetLineCalc/MATLAB Function1 ==
  data: HWASts input uint8 size=1; HWALeLineValid output boolean size=1; RoadWidth input single size=1; LineValid input boolean size=1; LineC3 input single size=1; LineC2 input single size=1; LineC1 input single size=1; LineC0 input single size=1; LineRange input single size=1; LeLineValid input boolean size=1; LeLineC3 input single size=1; LeLineC2 input single size=1; LeLineC1 input single size=1; LeLineC0 input single size=1; LeLineRange input single size=1; RiLineValid input boolean size=1; RiLineC3 input single size=1; RiLineC2 input single size=1; RiLineC1 input single size=1; RiLineC0 input single size=1; RiLineRange input single size=1; HWALeLineC3 output single size=1; HWALeLineC2 output single size=1; HWALeLineC1 output single size=1; HWALeLineC0 output single size=1; HWALeLineRange output single size=1; LeLineVirtual_b output boolean size=1; HWARiLineValid output boolean size=1; HWARiLineC3 output single size=1; HWARiLineC2 output single size=1; HWARiLineC1 output single size=1; HWARiLineC0 output single size=1; HWARiLineRange output single size=1; RiLineVirtual_b output boolean size=1
function [HWALeLineValid,HWALeLineC3,HWALeLineC2,HWALeLineC1,HWALeLineC0,HWALeLineRange,LeLineVirtual_b,...
    HWARiLineValid,HWARiLineC3,HWARiLineC2,HWARiLineC1,HWARiLineC0,HWARiLineRange,RiLineVirtual_b]...
    = LineAddCalc(HWASts,RoadWidth,LineValid,LineC3,LineC2,LineC1,LineC0,LineRange,...
    LeLineValid,LeLineC3,LeLineC2,LeLineC1,LeLineC0,LeLineRange,...
    RiLineValid,RiLineC3,RiLineC2,RiLineC1,RiLineC0,RiLineRange)

if LeLineValid==true||HWASts~=3
    HWALeLineValid = LeLineValid;
    HWALeLineC3 = LeLineC3;
    HWALeLineC2 = LeLineC2;
    HWALeLineC1 = LeLineC1;
    HWALeLineC0 = LeLineC0;
    HWALeLineRange = LeLineRange;
    LeLineVirtual_b = false;
else
    HWALeLineValid = false;
    HWALeLineC3 = LineC3;
    HWALeLineC2 = LineC2;
    HWALeLineC1 = LineC1;
    HWALeLineC0 = LineC0 + RoadWidth;
    HWALeLineRange = LineRange;
    LeLineVirtual_b = true;
end

if RiLineValid==true||HWASts~=3
    HWARiLineValid = RiLineValid;
    HWARiLineC3 = RiLineC3;
    HWARiLineC2 = RiLineC2;
    HWARiLineC1 = RiLineC1;
    HWARiLineC0 = RiLineC0;
    HWARiLineRange = RiLineRange;
    RiLineVirtual_b = false;
else
    HWARiLineValid = false;
    HWARiLineC3 = LineC3;
    HWARiLineC2 = LineC2;
    HWARiLineC1 = LineC1;
    HWARiLineC0 = LineC0 - RoadWidth;
    HWARiLineRange = LineRange;
    RiLineVirtual_b = true;
end

== matlab function PubIfDecisionLSM_MDL/Subsystem1/TargetLineCalc_20ms/TargetLineCalc/MATLAB Function2 ==
  data: LH1Wij input; LH2Wij input; LH1_Valid output; LH2_Valid output; Wij_state output; kap input; preDis input; VisLineA3 input; VisLineA2 input; VisLineA1 input; VisLineA0 input
function [LH1_Valid,LH2_Valid,Wij_state] = fcn(LH1Wij,LH2Wij,...
    kap,preDis,VisLineA3,VisLineA2,VisLineA1,VisLineA0)

LH1_Valid = false;
LH2_Valid = false;
Wij_state = uint8(0);

dy_pre = 0.5*kap*preDis^2;
Curature2_pre = VisLineA1(2) + 2*VisLineA2(2)*preDis + 3*VisLineA3(2)*(preDis^2);
Curature3_pre = VisLineA1(3) + 2*VisLineA2(3)*preDis + 3*VisLineA3(3)*(preDis^2);
dy2 = (VisLineA0(2) + VisLineA1(2)*preDis + VisLineA2(2)*(preDis^2) + VisLineA3(2)*(preDis^3) - dy_pre)/sqrt(Curature2_pre^2+single(1));
dy3 = (VisLineA0(3) + VisLineA1(3)*preDis + VisLineA2(3)*(preDis^2) + VisLineA3(3)*(preDis^3) - dy_pre)/sqrt(Curature3_pre^2+single(1));
RoadWidth_Cur = VisLineA0(2)-VisLineA0(3);

if LH1Wij >= 0.3 && LH2Wij >= 0.3  %置信度都比较高
%     if LeftLightReq
%        LH1_Valid = true;
%        Wij_state = uint8(1);
%     elseif RightLightReq  %开启右转向
%         LH2_Valid = true;
%         Wij_state = uint8(2);
%     elseif StubValid>0 && StubStartDis<60 && (Direction==3 || Direction==1)  % 导航向左
%                 LH1_Valid = true;
%                 Wij_state = uint8(3);
%     elseif StubValid>0 && StubStartDis<60 && (Direction==4 || Direction==2)  % 导航向右
%                 LH2_Valid = true;
%                 Wij_state = uint8(4);
    
    if RoadWidth_Cur-(dy2-dy3)>0.5  || dy2-dy3-RoadWidth_Cur>0.5 ||...
            abs(VisLineA0(2) - VisLineA0(3))>4.2 ||...
            abs(VisLineA0(2) - VisLineA0(3))<2.6     %没方向，有分叉或过宽、过窄
        if LH1Wij >= LH2Wij
            LH1_Valid = true;
            Wij_state = uint8(3);
        else
            LH2_Valid = true;
            Wij_state = uint8(4);
        end
    else  %没方向，没分叉
        LH1_Valid = true;
        LH2_Valid = true;
        Wij_state = uint8(5);
    end
    
elseif LH1Wij >= 0.3 
    LH1_Valid = true;
    Wij_state = uint8(1);
elseif LH2Wij >= 0.3
    LH2_Valid = true;
    Wij_state = uint8(2);
end

== matlab function PubIfDecisionLSM_MDL/Subsystem1/TargetLineCalc_20ms/TargetLineCalc/MATLAB Function3 ==
  data: LH1_Valid input; LH2_Valid input; CentLineValid output; VisLineA3 input; VisLineA2 input; VisLineA1 input; VisLineA0 input; VisLineR input; RoadWidth input; CentLineC3 output; CentLineC2 output; CentLineC1 output; CentLineC0 output; CentLineRange output; CentLineReliable output; Line_State output; LH1Wij input; LH2Wij input
function [CentLineValid,CentLineC3,CentLineC2,CentLineC1,CentLineC0,CentLineRange,CentLineReliable,Line_State] = ...
    VisFilter(LH1_Valid,LH2_Valid,...
    VisLineA3,VisLineA2,VisLineA1,VisLineA0,VisLineR,RoadWidth,LH1Wij,LH2Wij)

CentLineValid = false;
CentLineC0 = single(0);
CentLineC1 = single(0);
CentLineC2 = single(0);
CentLineC3 = single(0);
CentLineRange = single(0);
CentLineReliable = single(0);
Line_State = uint8(0);

if (LH1_Valid) && (LH2_Valid)
    Range_Error = VisLineR(2) - VisLineR(3);
    LH1_Offset = single(0.5);
    LH2_Offset = single(0.5);
    if Range_Error>10 || Range_Error<-10
        LH1_Offset = 0.5+min(0.5,Range_Error*0.01);
        LH2_Offset = 1-LH1_Offset;
    end
    CentLineValid = true;
    CentLineC0 = 0.5*(VisLineA0(2) + VisLineA0(3));
    CentLineC1 = LH1_Offset*VisLineA1(2) + LH2_Offset*VisLineA1(3);
    CentLineC2 = LH1_Offset*VisLineA2(2) + LH2_Offset*VisLineA2(3);
    CentLineC3 = LH1_Offset*VisLineA3(2) + LH2_Offset*VisLineA3(3);
    CentLineRange = max(VisLineR(2),VisLineR(3));
    CentLineReliable = 0.5*(LH1Wij+LH2Wij);
    Line_State = uint8(1);
elseif LH1_Valid
    CentLineValid = true;
    CentLineC0 = VisLineA0(2)-0.5*RoadWidth*sqrt(1+VisLineA1(2)*VisLineA1(2));
    CentLineC1 = VisLineA1(2);
    CentLineC2 = VisLineA2(2);
    CentLineC3 = VisLineA3(2);
    CentLineRange = VisLineR(2);
    CentLineReliable = LH1Wij;
    Line_State = uint8(2);
elseif LH2_Valid
    CentLineValid = true;
    CentLineC0 = VisLineA0(3)+0.5*RoadWidth*sqrt(1+VisLineA1(3)*VisLineA1(3));
    CentLineC1 = VisLineA1(3);
    CentLineC2 = VisLineA2(3);
    CentLineC3 = VisLineA3(3);
    CentLineRange = VisLineR(3);
    CentLineReliable = LH2Wij;
    Line_State = uint8(3);
end
